simulink library "inp"  (R2021b)
settings: Solver=VariableStepAuto  StartTime=0.0  StopTime=10.0  RelTol=1e-3
undefined symbols (not defined in the file): C_TASK_5MS_S, FALSE, KINP_AcoreReadyToSlp_flg_ovrdflg, KINP_AcoreReadyToSlp_flg_ovrdval, KINP_AllowMovThd_OTA_enum_ovrdflg, KINP_AllowMovThd_OTA_enum_ovrdval, KINP_APSAngleTarget_Deg_ovrdflg, KINP_APSAngleTarget_Deg_ovrdval, KINP_APSDecReq_mps2_ovrdflg, KINP_APSDecReq_mps2_ovrdval, KINP_APSDecReqA_flg_ovrdflg, KINP_APSDecReqA_flg_ovrdval, KINP_APSDFLL_cm_ovrdflg, KINP_APSDFLL_cm_ovrdval, KINP_APSDFLR_cm_ovrdflg, KINP_APSDFLR_cm_ovrdval, KINP_APSDRLL_cm_ovrdflg, KINP_APSDRLL_cm_ovrdval, KINP_APSDRLR_cm_ovrdflg, KINP_APSDRLR_cm_ovrdval, KINP_APSExitCondition_enum_ovrdflg, KINP_APSExitCondition_enum_ovrdval, KINP_APSHWVer_enum_ovrdflg, KINP_APSHWVer_enum_ovrdval, KINP_APSProgressPCT_pct_ovrdflg, KINP_APSProgressPCT_pct_ovrdval, KINP_APSReq_enum_ovrdflg, KINP_APSReq_enum_ovrdval, KINP_APSRQDisplay_enum_ovrdflg, KINP_APSRQDisplay_enum_ovrdval, KINP_APSRqEPASCtrl_flg_ovrdflg, KINP_APSRqEPASCtrl_flg_ovrdval, KINP_APSShiftPosnReq_enum_ovrdval, KINP_APSShiftPosnReq_enum_ovrflg, KINP_APSSpeedCMD_kph_ovrdval, KINP_APSSpeedCMD_kph_ovrflg, KINP_APSStaSystem_enum_ovrdflg, KINP_APSStaSystem_enum_ovrdval, KINP_APSSWVer_enum_ovrdflg, KINP_APSSWVer_enum_ovrdval, KINP_APSVMCReqA_flg_ovrdval, KINP_APSVMCReqA_flg_ovrflg, KINP_APSVRqEPASCtrl_flg_ovrdflg, KINP_APSVRqEPASCtrl_flg_ovrdval, KINP_AuxBattVolmV_mV_ovrdflg, KINP_AuxBattVolmV_mV_ovrdval, KINP_CAASSta_enum_ovrdflg, KINP_CAASSta_enum_ovrdval, KINP_CAASVMCReqA_flg_ovrdval, KINP_CAASVMCReqA_flg_ovrflg, KINP_Chime_enum_ovrdflg, KINP_Chime_enum_ovrdval, KINP_ClearDTCcmd_flg_ovrdflg, KINP_ClearDTCcmd_flg_ovrdval, KINP_EvccAplusPwrUpReq_flg_ovrdflg, KINP_EvccAplusPwrUpReq_flg_ovrdval, KINP_LFID_raw_ovrdval, KINP_LFID_raw_ovrflg, KINP_LRID_raw_ovrdval, KINP_MemOffsetAccX_raw16_ovrdflg ... (+118)
libraries: FVT_lib x595, hcu_lib x1
(part 5 of 27)

== system inp/INP/CAN3/CommunicationCheck ==
  BHAL_outputs : Inport
  CANMsgInvalidBMS1 : FVT_lib/inp/CAN_Msg_Validity_Process_template  SystemSampleTime=-1  VariantActivationTime=update diagram  Latency=0  AutoFrameSizeCalculation=off
      link override debdec: Value=KINP_CANMsgInvalidBMS1_flg_debdec
      link override debinc: Value=KINP_CANMsgInvalidBMS1_flg_debinc
      link override deblim: Value=KINP_CANMsgInvalidBMS1_flg_deblim
      link override inverse: Value=KINP_CANMsgInvalidBMS1_flg_inverse
      link override ovrdflg: Value=KINP_CANMsgInvalidBMS1_flg_ovrdflg
      link override ovrdval: Value=KINP_CANMsgInvalidBMS1_flg_ovrdval
      link override srvcflg: Value=KINP_CANMsgInvalidBMS1_flg_srvcflg
      link override srvcval: Value=KINP_CANMsgInvalidBMS1_flg_srvcval
  CANMsgInvalidBMS2 : FVT_lib/inp/CAN_Msg_Validity_Process_template  SystemSampleTime=-1  VariantActivationTime=update diagram  Latency=0  AutoFrameSizeCalculation=off
      link override debdec: Value=KINP_CANMsgInvalidBMS2_flg_debdec
      link override debinc: Value=KINP_CANMsgInvalidBMS2_flg_debinc
      link override deblim: Value=KINP_CANMsgInvalidBMS2_flg_deblim
      link override inverse: Value=KINP_CANMsgInvalidBMS2_flg_inverse
      link override ovrdflg: Value=KINP_CANMsgInvalidBMS2_flg_ovrdflg
      link override ovrdval: Value=KINP_CANMsgInvalidBMS2_flg_ovrdval
      link override srvcflg: Value=KINP_CANMsgInvalidBMS2_flg_srvcflg
      link override srvcval: Value=KINP_CANMsgInvalidBMS2_flg_srvcval
  CANMsgInvalidBMS3 : FVT_lib/inp/CAN_Msg_Validity_Process_template  SystemSampleTime=-1  VariantActivationTime=update diagram  Latency=0  AutoFrameSizeCalculation=off
      link override debdec: Value=KINP_CANMsgInvalidBMS3_flg_debdec
      link override debinc: Value=KINP_CANMsgInvalidBMS3_flg_debinc
      link override deblim: Value=KINP_CANMsgInvalidBMS3_flg_deblim
      link override inverse: Value=KINP_CANMsgInvalidBMS3_flg_inverse
      link override ovrdflg: Value=KINP_CANMsgInvalidBMS3_flg_ovrdflg
      link override ovrdval: Value=KINP_CANMsgInvalidBMS3_flg_ovrdval
      link override srvcflg: Value=KINP_CANMsgInvalidBMS3_flg_srvcflg
      link override srvcval: Value=KINP_CANMsgInvalidBMS3_flg_srvcval
  CANMsgInvalidBMS4 : FVT_lib/inp/CAN_Msg_Validity_Process_template  SystemSampleTime=-1  VariantActivationTime=update diagram  Latency=0  AutoFrameSizeCalculation=off
      link override debdec: Value=KINP_CANMsgInvalidBMS4_flg_debdec
      link override debinc: Value=KINP_CANMsgInvalidBMS4_flg_debinc
      link override deblim: Value=KINP_CANMsgInvalidBMS4_flg_deblim
      link override inverse: Value=KINP_CANMsgInvalidBMS4_flg_inverse
      link override ovrdflg: Value=KINP_CANMsgInvalidBMS4_flg_ovrdflg
      link override ovrdval: Value=KINP_CANMsgInvalidBMS4_flg_ovrdval
      link override srvcflg: Value=KINP_CANMsgInvalidBMS4_flg_srvcflg
      link override srvcval: Value=KINP_CANMsgInvalidBMS4_flg_srvcval
  CANMsgInvalidBMS6 : FVT_lib/inp/CAN_Msg_Validity_Process_template  SystemSampleTime=-1  VariantActivationTime=update diagram  Latency=0  AutoFrameSizeCalculation=off
      link override debdec: Value=KINP_CANMsgInvalidBMS6_flg_debdec
      link override debinc: Value=KINP_CANMsgInvalidBMS6_flg_debinc
      link override deblim: Value=KINP_CANMsgInvalidBMS6_flg_deblim
      link override inverse: Value=KINP_CANMsgInvalidBMS6_flg_inverse
      link override ovrdflg: Value=KINP_CANMsgInvalidBMS6_flg_ovrdflg
      link override ovrdval: Value=KINP_CANMsgInvalidBMS6_flg_ovrdval
      link override srvcflg: Value=KINP_CANMsgInvalidBMS6_flg_srvcflg
      link override srvcval: Value=KINP_CANMsgInvalidBMS6_flg_srvcval
  CANMsgInvalidBMS7 : FVT_lib/inp/CAN_Msg_Validity_Process_template  SystemSampleTime=-1  VariantActivationTime=update diagram  Latency=0  AutoFrameSizeCalculation=off
      link override debdec: Value=KINP_CANMsgInvalidBMS7_flg_debdec
      link override debinc: Value=KINP_CANMsgInvalidBMS7_flg_debinc
      link override deblim: Value=KINP_CANMsgInvalidBMS7_flg_deblim
      link override inverse: Value=KINP_CANMsgInvalidBMS7_flg_inverse
      link override ovrdflg: Value=KINP_CANMsgInvalidBMS7_flg_ovrdflg
      link override ovrdval: Value=KINP_CANMsgInvalidBMS7_flg_ovrdval
      link override srvcflg: Value=KINP_CANMsgInvalidBMS7_flg_srvcflg
      link override srvcval: Value=KINP_CANMsgInvalidBMS7_flg_srvcval
  CANMsgInvalidCCU1 : FVT_lib/inp/CAN_Msg_Validity_Process_template  SystemSampleTime=-1  VariantActivationTime=update diagram  Latency=0  AutoFrameSizeCalculation=off
      link override debdec: Value=KINP_CANMsgInvalidCCU1_flg_debdec
      link override debinc: Value=KINP_CANMsgInvalidCCU1_flg_debinc
      link override deblim: Value=KINP_CANMsgInvalidCCU1_flg_deblim
      link override inverse: Value=KINP_CANMsgInvalidCCU1_flg_inverse
      link override ovrdflg: Value=KINP_CANMsgInvalidCCU1_flg_ovrdflg
      link override ovrdval: Value=KINP_CANMsgInvalidCCU1_flg_ovrdval
      link override srvcflg: Value=KINP_CANMsgInvalidCCU1_flg_srvcflg
      link override srvcval: Value=KINP_CANMsgInvalidCCU1_flg_srvcval
  CANMsgInvalidCCU2 : FVT_lib/inp/CAN_Msg_Validity_Process_template  SystemSampleTime=-1  VariantActivationTime=update diagram  Latency=0  AutoFrameSizeCalculation=off
      link override debdec: Value=KINP_CANMsgInvalidCCU2_flg_debdec
      link override debinc: Value=KINP_CANMsgInvalidCCU2_flg_debinc
      link override deblim: Value=KINP_CANMsgInvalidCCU2_flg_deblim
      link override inverse: Value=KINP_CANMsgInvalidCCU2_flg_inverse
      link override ovrdflg: Value=KINP_CANMsgInvalidCCU2_flg_ovrdflg
      link override ovrdval: Value=KINP_CANMsgInvalidCCU2_flg_ovrdval
      link override srvcflg: Value=KINP_CANMsgInvalidCCU2_flg_srvcflg
      link override srvcval: Value=KINP_CANMsgInvalidCCU2_flg_srvcval
  CANMsgInvalidCCU4 : FVT_lib/inp/CAN_Msg_Validity_Process_template  SystemSampleTime=-1  VariantActivationTime=update diagram  Latency=0  AutoFrameSizeCalculation=off
      link override debdec: Value=KINP_CANMsgInvalidCCU4_flg_debdec
      link override debinc: Value=KINP_CANMsgInvalidCCU4_flg_debinc
      link override deblim: Value=KINP_CANMsgInvalidCCU4_flg_deblim
      link override inverse: Value=KINP_CANMsgInvalidCCU4_flg_inverse
      link override ovrdflg: Value=KINP_CANMsgInvalidCCU4_flg_ovrdflg
      link override ovrdval: Value=KINP_CANMsgInvalidCCU4_flg_ovrdval
      link override srvcflg: Value=KINP_CANMsgInvalidCCU4_flg_srvcflg
      link override srvcval: Value=KINP_CANMsgInvalidCCU4_flg_srvcval
  CANMsgInvalidMCUF1 : FVT_lib/inp/CAN_Msg_Validity_Process_template  SystemSampleTime=-1  VariantActivationTime=update diagram  Latency=0  AutoFrameSizeCalculation=off
      link override debdec: Value=KINP_CANMsgInvalidMCUF1_flg_debdec
      link override debinc: Value=KINP_CANMsgInvalidMCUF1_flg_debinc
      link override deblim: Value=KINP_CANMsgInvalidMCUF1_flg_deblim
      link override inverse: Value=KINP_CANMsgInvalidMCUF1_flg_inverse
      link override ovrdflg: Value=KINP_CANMsgInvalidMCUF1_flg_ovrdflg
      link override ovrdval: Value=KINP_CANMsgInvalidMCUF1_flg_ovrdval
      link override srvcflg: Value=KINP_CANMsgInvalidMCUF1_flg_srvcflg
      link override srvcval: Value=KINP_CANMsgInvalidMCUF1_flg_srvcval
  CANMsgInvalidMCUF2 : FVT_lib/inp/CAN_Msg_Validity_Process_template  SystemSampleTime=-1  VariantActivationTime=update diagram  Latency=0  AutoFrameSizeCalculation=off
      link override debdec: Value=KINP_CANMsgInvalidMCUF2_flg_debdec
      link override debinc: Value=KINP_CANMsgInvalidMCUF2_flg_debinc
      link override deblim: Value=KINP_CANMsgInvalidMCUF2_flg_deblim
      link override inverse: Value=KINP_CANMsgInvalidMCUF2_flg_inverse
      link override ovrdflg: Value=KINP_CANMsgInvalidMCUF2_flg_ovrdflg
      link override ovrdval: Value=KINP_CANMsgInvalidMCUF2_flg_ovrdval
      link override srvcflg: Value=KINP_CANMsgInvalidMCUF2_flg_srvcflg
      link override srvcval: Value=KINP_CANMsgInvalidMCUF2_flg_srvcval
  CANMsgInvalidMCUR1 : FVT_lib/inp/CAN_Msg_Validity_Process_template  SystemSampleTime=-1  VariantActivationTime=update diagram  Latency=0  AutoFrameSizeCalculation=off
      link override debdec: Value=KINP_CANMsgInvalidMCUR1_flg_debdec
      link override debinc: Value=KINP_CANMsgInvalidMCUR1_flg_debinc
      link override deblim: Value=KINP_CANMsgInvalidMCUR1_flg_deblim
      link override inverse: Value=KINP_CANMsgInvalidMCUR1_flg_inverse
      link override ovrdflg: Value=KINP_CANMsgInvalidMCUR1_flg_ovrdflg
      link override ovrdval: Value=KINP_CANMsgInvalidMCUR1_flg_ovrdval
      link override srvcflg: Value=KINP_CANMsgInvalidMCUR1_flg_srvcflg
      link override srvcval: Value=KINP_CANMsgInvalidMCUR1_flg_srvcval
  CANMsgInvalidMCUR2 : FVT_lib/inp/CAN_Msg_Validity_Process_template  SystemSampleTime=-1  VariantActivationTime=update diagram  Latency=0  AutoFrameSizeCalculation=off
      link override debdec: Value=KINP_CANMsgInvalidMCUR2_flg_debdec
      link override debinc: Value=KINP_CANMsgInvalidMCUR2_flg_debinc
      link override deblim: Value=KINP_CANMsgInvalidMCUR2_flg_deblim
      link override inverse: Value=KINP_CANMsgInvalidMCUR2_flg_inverse
      link override ovrdflg: Value=KINP_CANMsgInvalidMCUR2_flg_ovrdflg
      link override ovrdval: Value=KINP_CANMsgInvalidMCUR2_flg_ovrdval
      link override srvcflg: Value=KINP_CANMsgInvalidMCUR2_flg_srvcflg
      link override srvcval: Value=KINP_CANMsgInvalidMCUR2_flg_srvcval
  CANMsgInvalidShifter1 : FVT_lib/inp/CAN_Msg_Validity_Process_template  SystemSampleTime=-1  VariantActivationTime=update diagram  Latency=0  AutoFrameSizeCalculation=off
      link override debdec: Value=KINP_CANMsgInvalidShifter1_flg_debdec
      link override debinc: Value=KINP_CANMsgInvalidShifter1_flg_debinc
      link override deblim: Value=KINP_CANMsgInvalidShifter1_flg_deblim
      link override inverse: Value=KINP_CANMsgInvalidShifter1_flg_inverse
      link override ovrdflg: Value=KINP_CANMsgInvalidShifter1_flg_ovrdflg
      link override ovrdval: Value=KINP_CANMsgInvalidShifter1_flg_ovrdval
      link override srvcflg: Value=KINP_CANMsgInvalidShifter1_flg_srvcflg
      link override srvcval: Value=KINP_CANMsgInvalidShifter1_flg_srvcval
  bus_creator : BusCreator  Inputs=14
  bus_selector : BusSelector  OutputSignals=VHAL_CANMsgInvalidBMS1_flg,VHAL_CANMsgInvalidBMS2_flg,VHAL_CANMsgInvalidBMS3_flg,VHAL_CANMsgInvalidBMS4_flg,VHAL_CANMsgInvalidBMS6_flg,VHAL_CANMsgInvalidBMS7_flg,VHAL_CANMsgInvalidCCU1_flg,VHAL_CANMsgInvalidCCU2_flg,VHAL_CANMsgInvalidCCU4_flg,VHAL_CANMsgInvalidMCUF1_flg,VHAL_CANMsgInvalidMCUF2_flg,VHAL_CANMsgInvalidMCUR1_flg,VHAL_CANMsgInvalidMCUR2_flg,VHAL_CANMsgInvalidShifter1_flg
  not{1..14} (14 alike) : Logic  Operator=NOT  AllPortsSameDT=off  OutDataTypeStr=boolean
  inp_CanValid_bus : Outport
  wires:
  BHAL_outputs/1 -> [BHAL_outputs]
  bus_selector/1 -> CANMsgInvalidBMS1/1  "<VHAL_CANMsgInvalidBMS1_flg>"
  CANMsgInvalidBMS1/1 -> not1/1
  not1/1 -> bus_creator/1  "VINP_CANMsgValidBMS1_flg"
  bus_selector/2 -> CANMsgInvalidBMS2/1  "<VHAL_CANMsgInvalidBMS2_flg>"
  CANMsgInvalidBMS2/1 -> not2/1
  not2/1 -> bus_creator/2  "VINP_CANMsgValidBMS2_flg"
  bus_selector/3 -> CANMsgInvalidBMS3/1  "<VHAL_CANMsgInvalidBMS3_flg>"
  CANMsgInvalidBMS3/1 -> not3/1
  not3/1 -> bus_creator/3  "VINP_CANMsgValidBMS3_flg"
  bus_selector/4 -> CANMsgInvalidBMS4/1  "<VHAL_CANMsgInvalidBMS4_flg>"
  CANMsgInvalidBMS4/1 -> not4/1
  not4/1 -> bus_creator/4  "VINP_CANMsgValidBMS4_flg"
  bus_selector/5 -> CANMsgInvalidBMS6/1  "<VHAL_CANMsgInvalidBMS6_flg>"
  CANMsgInvalidBMS6/1 -> not5/1
  not5/1 -> bus_creator/5  "VINP_CANMsgValidBMS6_flg"
  bus_selector/6 -> CANMsgInvalidBMS7/1  "<VHAL_CANMsgInvalidBMS7_flg>"
  CANMsgInvalidBMS7/1 -> not6/1
  not6/1 -> bus_creator/6  "VINP_CANMsgValidBMS7_flg"
  bus_selector/7 -> CANMsgInvalidCCU1/1  "<VHAL_CANMsgInvalidCCU1_flg>"
  CANMsgInvalidCCU1/1 -> not7/1
  not7/1 -> bus_creator/7  "VINP_CANMsgValidCCU1_flg"
  bus_selector/8 -> CANMsgInvalidCCU2/1  "<VHAL_CANMsgInvalidCCU2_flg>"
  CANMsgInvalidCCU2/1 -> not8/1
  not8/1 -> bus_creator/8  "VINP_CANMsgValidCCU2_flg"
  bus_selector/9 -> CANMsgInvalidCCU4/1  "<VHAL_CANMsgInvalidCCU4_flg>"
  CANMsgInvalidCCU4/1 -> not9/1
  not9/1 -> bus_creator/9  "VINP_CANMsgValidCCU4_flg"
  bus_selector/10 -> CANMsgInvalidMCUF1/1  "<VHAL_CANMsgInvalidMCUF1_flg>"
  CANMsgInvalidMCUF1/1 -> not10/1
  not10/1 -> bus_creator/10  "VINP_CANMsgValidMCUF1_flg"
  bus_selector/11 -> CANMsgInvalidMCUF2/1  "<VHAL_CANMsgInvalidMCUF2_flg>"
  CANMsgInvalidMCUF2/1 -> not11/1
  not11/1 -> bus_creator/11  "VINP_CANMsgValidMCUF2_flg"
  bus_selector/12 -> CANMsgInvalidMCUR1/1  "<VHAL_CANMsgInvalidMCUR1_flg>"
  CANMsgInvalidMCUR1/1 -> not12/1
  not12/1 -> bus_creator/12  "VINP_CANMsgValidMCUR1_flg"
  bus_selector/13 -> CANMsgInvalidMCUR2/1  "<VHAL_CANMsgInvalidMCUR2_flg>"
  CANMsgInvalidMCUR2/1 -> not13/1
  not13/1 -> bus_creator/13  "VINP_CANMsgValidMCUR2_flg"
  bus_selector/14 -> CANMsgInvalidShifter1/1  "<VHAL_CANMsgInvalidShifter1_flg>"
  CANMsgInvalidShifter1/1 -> not14/1
  not14/1 -> bus_creator/14  "VINP_CANMsgValidShifter1_flg"
  [BHAL_outputs] -> bus_selector/1
  bus_creator/1 -> inp_CanValid_bus/1

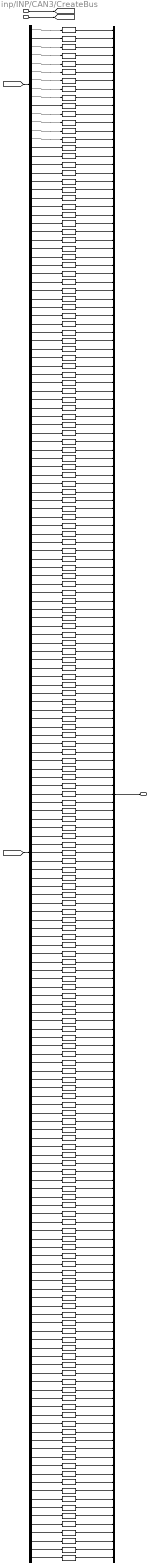
== system inp/INP/CAN3/CreateBus ==
  inp_CanValid_bus : Inport
  inp_Hal_bus : Inport  Port=2
  UnitConverter_{1..16,51..52,55..63,66..67,70,72..74,82,84..85,87,89,93,95..96,103..107,116..117,119..121,141..142,144..146,155..156,158..160,179..180} (63 alike) : DataTypeConversion  OutDataTypeStr=boolean
  UnitConverter_{17..18,47..50,53..54,64..65,68..69,71,75,78,81,83,86,88,94,98..100,109,111..112,118,122,130,133..136,139..140,143,148,150..151,157,161,171..174,177..178,181..183} (50 alike) : DataTypeConversion  OutDataTypeStr=uint8
  UnitConverter_{19..46,76..77,79..80,90..92,97,101..102,108,110,113..115,123..129,131..132,137..138,147,149,152..154,162..170,175..176} (70 alike) : DataTypeConversion  OutDataTypeStr=single
  bus_creator : BusCreator  Inputs=183
  bus_selector : BusSelector  OutputSignals=VINP_CANMsgValidBMS1_flg,VINP_CANMsgValidBMS2_flg,VINP_CANMsgValidBMS3_flg,VINP_CANMsgValidBMS4_flg,VINP_CANMsgValidBMS6_flg,VINP_CANMsgValidBMS7_flg,VINP_CANMsgValidCCU1_flg,VINP_CANMsgValidCCU2_flg,VINP_CANMsgValidCCU4_flg,VINP_CANMsgValidMCUF1_flg,VINP_CANMsgValidMCUF2_flg,VINP_CANMsgValidMCUR1_flg,VINP_CANMsgValidMCUR2_flg,VINP_CANMsgValidShifter1_flg
  bus_selector_1 : BusSelector  OutputSignals=VINP_BMS1CSErr_flg,VINP_BMS1RCErr_flg,VINP_BMSChckSum1_enum,VINP_BMSRolCnct1_enum,VINP_HVBPwrAvailChrg_kW,VINP_HVBPwrAvailChrg30_kW,VINP_HVBPwrAvailChrg60_kW,VINP_HVBPwrAvailDchrg_kW,VINP_HVBPwrAvailDchrg30_kW,VINP_HVBPwrAvailDchrg60_kW,VINP_HVInVolt_V,VINP_LVBattDet12V_V,VINP_OBCDCCurLm_A,VINP_OBCDCVoltLm_V,VINP_ACChrgCurrDis_A,VINP_HVBChrgPwr_kWh,VINP_HVBChrgPwrTotal_kWh,VINP_HVBDrvPwr_kWh,VINP_HVBDrvPwrTotal_kWh,VINP_HVBFullChrgPwr_kWh,VINP_HVBIsoImpedenceN_Megaohm,VINP_HVBIsoImpedenceP_Megaohm,VINP_HVBSOH_pct,VINP_HVBattPackVolt_V,VINP_HVBattSOC_pct,VINP_HVBattSOCDis_pct,VINP_RemainChrgTime_min,VINP_CellTempAvg_C,VINP_HVBCellVoltMax_mV,VINP_HVBCellVoltMin_mV,VINP_HVBMTempMax_C,VINP_HVBMTempMin_C,VINP_MaxCellTempNum_enum,VINP_MaxCellVoltNum_enum,VINP_MinCellTempNum_enum,VINP_MinCellVoltNum_enum,VINP_BMS6CSErr_flg,VINP_BMS6RCErr_flg,VINP_BMSChckSum_enum,VINP_BMSRolCnct_enum,VINP_BMSREADY_flg,VINP_BMSWarn1_flg,VINP_BMSWarn2_flg,VINP_BMSWarn3_flg,VINP_BMSWarn4_flg,VINP_BMSWarn5_flg,VINP_BMSWarn6_flg,VINP_BMSWarn7_flg,VINP_BMSWarn8_flg,VINP_ChrgPlugSta_enum,VINP_ExtChrgSta_enum,VINP_HVBContactorSta_flg,VINP_HVBHVILErr_flg,VINP_HVBPreheatPrecoolSta_enum,VINP_HVBattReady4Pre_enum,VINP_HVILSta_flg,VINP_V2LSta_enum,VINP_HVBattErr_flg,VINP_CCU1CSErr_flg,VINP_CCU1RCErr_flg,VINP_CSCCU1_enum,VINP_DCDCAuxVolt_V,VINP_DCDCInVoltInf_V,VINP_DCDCPreCompleted_enum,VINP_OBCDCCurrInf_A,VINP_OBCDCVoltInf_V,VINP_OBCPreCompleted_enum,VINP_OBCWakeup4Plugin_flg,VINP_RCCCU1_enum,VINP_CCU2CSErr_flg,VINP_CCU2RCErr_flg,VINP_CSCCU2_enum,VINP_DCDCEnaSta_flg,VINP_DCDCFaultSta_enum,VINP_DCDCReady4Pre_flg,VINP_DCDCTemp_C,VINP_OBCACCurrInf_A,VINP_OBCACVoltInf_V,VINP_OBCEnaSta_flg,VINP_OBCFaultSta_enum,VINP_OBCPluginSta_flg,VINP_OBCReady4Pre_flg,VINP_OBCTemp_C,VINP_OBCV2LSta_enum,VINP_OBCACCurLim_enum,VINP_RCCCU2_enum,VINP_DCDCAuxCur_A,VINP_DCDCHVCur_A,VINP_MCUF1CSErr_flg,VINP_MCUF1RCErr_flg,VINP_FrActvDmpDisabSta_flg,VINP_FrEDUDrtSta_flg,VINP_FrEDUOpratingSta_flg,VINP_FrEDURealTMTq_Nm,VINP_FrEDURotateDirction_enum,VINP_FrEDUTqReqFbk_Nm,VINP_FrMCU1Chksum_enum,VINP_FrMCU1RolCnt_enum,VINP_FrMCUBAT_V,VINP_FrMCUDCBusCurr_A,VINP_FrMCUDCBusVolt_V,VINP_FrMCUDischrgSta_flg,VINP_FrMCUEnaSta_flg,VINP_FrMCUErr_enum,VINP_FrMCUIGNsta_flg,VINP_FrMCUReady_flg,VINP_FrMCUReady4Pre_flg,VINP_FrMCUSysSta_enum,VINP_FrMCUTemp_C,VINP_FrMotorAvailTq_Nm,VINP_FrRegenAvailTq_Nm,VINP_FrTMSpd_rpm,VINP_FrTMTemp_C,VINP_FrTMid_A,VINP_FrTMiq_A,VINP_MCUWarnF_enum,VINP_FrCoolanttempReq_C,VINP_FrEOPSpdSet_rpm,VINP_FrFailcode1_enum,VINP_FrFailcode2_enum,VINP_FrFailcodehistory1_enum,VINP_FrFailcodehistory2_enum,VINP_FrLLCTemp_C,VINP_FrLLCflowReq_Lpmin,VINP_FrMCUTempWarn_enum,VINP_FrTMTempWarn_enum,VINP_MCUR1CSErr_flg,VINP_MCUR1RCErr_flg,VINP_MCUWarnR_enum,VINP_RrActvDmpDisabSta_flg,VINP_RrEDUDrtSta_flg,VINP_RrEDUOpratingSta_flg,VINP_RrEDURealTMTq_Nm,VINP_RrEDURotateDirction_enum,VINP_RrEDUTqReqFbk_Nm,VINP_RrMCU1Chksum_enum,VINP_RrMCU1RolCnt_enum,VINP_RrMCUBAT_V,VINP_RrMCUDCBusCurr_A,VINP_RrMCUDCBusVolt_V,VINP_RrMCUDischrgSta_flg,VINP_RrMCUEnaSta_flg,VINP_RrMCUErr_enum,VINP_RrMCUIGNsta_flg,VINP_RrMCUReady_flg,VINP_RrMCUReady4Pre_flg,VINP_RrMCUSysSta_enum,VINP_RrMCUTemp_C,VINP_RrMotorAvailTq_Nm,VINP_RrRegenAvailTq_Nm,VINP_RrTMSpd_rpm,VINP_RrTMTemp_C,VINP_RrTMid_A,VINP_RrTMiq_A,VINP_RrCoolanttempReq_cnt,VINP_RrEOPSpdSet_rpm,VINP_RrFailcode1_enum,VINP_RrFailcode2_enum,VINP_RrFailcodehistory1_enum,VINP_RrFailcodehistory2_enum,VINP_RrLLCTemp_C,VINP_RrLLCflowReq_Lpmin,VINP_RrMCUTempWarn_enum,VINP_RrTMTempWarn_enum,VINP_Shifter1CSErr_flg,VINP_Shifter1RCErr_flg,VINP_ShifterCRC8_enum,VINP_ShifterHandleCmd_enum,VINP_ShifterRC_enum
  BINP_outputs : Outport
  wires:
  inp_CanValid_bus/1 -> [inp_CanValid_bus]
  inp_Hal_bus/1 -> [inp_Hal_bus]
  bus_selector/1 -> UnitConverter_1/1  "<VINP_CANMsgValidBMS1_flg>"
  UnitConverter_1/1 -> bus_creator/1  "VINP_CANMsgValidBMS1_flg"
  bus_selector/2 -> UnitConverter_2/1  "<VINP_CANMsgValidBMS2_flg>"
  UnitConverter_2/1 -> bus_creator/2  "VINP_CANMsgValidBMS2_flg"
  bus_selector/3 -> UnitConverter_3/1  "<VINP_CANMsgValidBMS3_flg>"
  UnitConverter_3/1 -> bus_creator/3  "VINP_CANMsgValidBMS3_flg"
  bus_selector/4 -> UnitConverter_4/1  "<VINP_CANMsgValidBMS4_flg>"
  UnitConverter_4/1 -> bus_creator/4  "VINP_CANMsgValidBMS4_flg"
  bus_selector/5 -> UnitConverter_5/1  "<VINP_CANMsgValidBMS6_flg>"
  UnitConverter_5/1 -> bus_creator/5  "VINP_CANMsgValidBMS6_flg"
  bus_selector/6 -> UnitConverter_6/1  "<VINP_CANMsgValidBMS7_flg>"
  UnitConverter_6/1 -> bus_creator/6  "VINP_CANMsgValidBMS7_flg"
  bus_selector/7 -> UnitConverter_7/1  "<VINP_CANMsgValidCCU1_flg>"
  UnitConverter_7/1 -> bus_creator/7  "VINP_CANMsgValidCCU1_flg"
  bus_selector/8 -> UnitConverter_8/1  "<VINP_CANMsgValidCCU2_flg>"
  UnitConverter_8/1 -> bus_creator/8  "VINP_CANMsgValidCCU2_flg"
  bus_selector/9 -> UnitConverter_9/1  "<VINP_CANMsgValidCCU4_flg>"
  UnitConverter_9/1 -> bus_creator/9  "VINP_CANMsgValidCCU4_flg"
  bus_selector/10 -> UnitConverter_10/1  "<VINP_CANMsgValidMCUF1_flg>"
  UnitConverter_10/1 -> bus_creator/10  "VINP_CANMsgValidMCUF1_flg"
  bus_selector/11 -> UnitConverter_11/1  "<VINP_CANMsgValidMCUF2_flg>"
  UnitConverter_11/1 -> bus_creator/11  "VINP_CANMsgValidMCUF2_flg"
  bus_selector/12 -> UnitConverter_12/1  "<VINP_CANMsgValidMCUR1_flg>"
  UnitConverter_12/1 -> bus_creator/12  "VINP_CANMsgValidMCUR1_flg"
  bus_selector/13 -> UnitConverter_13/1  "<VINP_CANMsgValidMCUR2_flg>"
  UnitConverter_13/1 -> bus_creator/13  "VINP_CANMsgValidMCUR2_flg"
  bus_selector/14 -> UnitConverter_14/1  "<VINP_CANMsgValidShifter1_flg>"
  UnitConverter_14/1 -> bus_creator/14  "VINP_CANMsgValidShifter1_flg"
  bus_selector_1/1 -> UnitConverter_15/1  "<VINP_BMS1CSErr_flg>"
  UnitConverter_15/1 -> bus_creator/15  "VINP_BMS1CSErr_flg"
  bus_selector_1/2 -> UnitConverter_16/1  "<VINP_BMS1RCErr_flg>"
  UnitConverter_16/1 -> bus_creator/16  "VINP_BMS1RCErr_flg"
  bus_selector_1/3 -> UnitConverter_17/1  "<VINP_BMSChckSum1_enum>"
  UnitConverter_17/1 -> bus_creator/17  "VINP_BMSChckSum1_enum"
  bus_selector_1/4 -> UnitConverter_18/1  "<VINP_BMSRolCnct1_enum>"
  UnitConverter_18/1 -> bus_creator/18  "VINP_BMSRolCnct1_enum"
  bus_selector_1/5 -> UnitConverter_19/1  "<VINP_HVBPwrAvailChrg_kW>"
  UnitConverter_19/1 -> bus_creator/19  "VINP_HVBPwrAvailChrg_kW"
  bus_selector_1/6 -> UnitConverter_20/1  "<VINP_HVBPwrAvailChrg30_kW>"
  UnitConverter_20/1 -> bus_creator/20  "VINP_HVBPwrAvailChrg30_kW"
  bus_selector_1/7 -> UnitConverter_21/1  "<VINP_HVBPwrAvailChrg60_kW>"
  UnitConverter_21/1 -> bus_creator/21  "VINP_HVBPwrAvailChrg60_kW"
  bus_selector_1/8 -> UnitConverter_22/1  "<VINP_HVBPwrAvailDchrg_kW>"
  UnitConverter_22/1 -> bus_creator/22  "VINP_HVBPwrAvailDchrg_kW"
  bus_selector_1/9 -> UnitConverter_23/1  "<VINP_HVBPwrAvailDchrg30_kW>"
  UnitConverter_23/1 -> bus_creator/23  "VINP_HVBPwrAvailDchrg30_kW"
  bus_selector_1/10 -> UnitConverter_24/1  "<VINP_HVBPwrAvailDchrg60_kW>"
  UnitConverter_24/1 -> bus_creator/24  "VINP_HVBPwrAvailDchrg60_kW"
  bus_selector_1/11 -> UnitConverter_25/1  "<VINP_HVInVolt_V>"
  UnitConverter_25/1 -> bus_creator/25  "VINP_HVInVolt_V"
  bus_selector_1/12 -> UnitConverter_26/1  "<VINP_LVBattDet12V_V>"
  UnitConverter_26/1 -> bus_creator/26  "VINP_LVBattDet12V_V"
  bus_selector_1/13 -> UnitConverter_27/1  "<VINP_OBCDCCurLm_A>"
  UnitConverter_27/1 -> bus_creator/27  "VINP_OBCDCCurLm_A"
  bus_selector_1/14 -> UnitConverter_28/1  "<VINP_OBCDCVoltLm_V>"
  UnitConverter_28/1 -> bus_creator/28  "VINP_OBCDCVoltLm_V"
  bus_selector_1/15 -> UnitConverter_29/1  "<VINP_ACChrgCurrDis_A>"
  UnitConverter_29/1 -> bus_creator/29  "VINP_ACChrgCurrDis_A"
  bus_selector_1/16 -> UnitConverter_30/1  "<VINP_HVBChrgPwr_kWh>"
  UnitConverter_30/1 -> bus_creator/30  "VINP_HVBChrgPwr_kWh"
  bus_selector_1/17 -> UnitConverter_31/1  "<VINP_HVBChrgPwrTotal_kWh>"
  UnitConverter_31/1 -> bus_creator/31  "VINP_HVBChrgPwrTotal_kWh"
  bus_selector_1/18 -> UnitConverter_32/1  "<VINP_HVBDrvPwr_kWh>"
  UnitConverter_32/1 -> bus_creator/32  "VINP_HVBDrvPwr_kWh"
  bus_selector_1/19 -> UnitConverter_33/1  "<VINP_HVBDrvPwrTotal_kWh>"
  UnitConverter_33/1 -> bus_creator/33  "VINP_HVBDrvPwrTotal_kWh"
  bus_selector_1/20 -> UnitConverter_34/1  "<VINP_HVBFullChrgPwr_kWh>"
  UnitConverter_34/1 -> bus_creator/34  "VINP_HVBFullChrgPwr_kWh"
  bus_selector_1/21 -> UnitConverter_35/1  "<VINP_HVBIsoImpedenceN_Megaohm>"
  UnitConverter_35/1 -> bus_creator/35  "VINP_HVBIsoImpedenceN_Megaohm"
  bus_selector_1/22 -> UnitConverter_36/1  "<VINP_HVBIsoImpedenceP_Megaohm>"
  UnitConverter_36/1 -> bus_creator/36  "VINP_HVBIsoImpedenceP_Megaohm"
  bus_selector_1/23 -> UnitConverter_37/1  "<VINP_HVBSOH_pct>"
  UnitConverter_37/1 -> bus_creator/37  "VINP_HVBSOH_pct"
  bus_selector_1/24 -> UnitConverter_38/1  "<VINP_HVBattPackVolt_V>"
  UnitConverter_38/1 -> bus_creator/38  "VINP_HVBattPackVolt_V"
  bus_selector_1/25 -> UnitConverter_39/1  "<VINP_HVBattSOC_pct>"
  UnitConverter_39/1 -> bus_creator/39  "VINP_HVBattSOC_pct"
  bus_selector_1/26 -> UnitConverter_40/1  "<VINP_HVBattSOCDis_pct>"
  UnitConverter_40/1 -> bus_creator/40  "VINP_HVBattSOCDis_pct"
  bus_selector_1/27 -> UnitConverter_41/1  "<VINP_RemainChrgTime_min>"
  UnitConverter_41/1 -> bus_creator/41  "VINP_RemainChrgTime_min"
  bus_selector_1/28 -> UnitConverter_42/1  "<VINP_CellTempAvg_C>"
  UnitConverter_42/1 -> bus_creator/42  "VINP_CellTempAvg_C"
  bus_selector_1/29 -> UnitConverter_43/1  "<VINP_HVBCellVoltMax_mV>"
  UnitConverter_43/1 -> bus_creator/43  "VINP_HVBCellVoltMax_mV"
  bus_selector_1/30 -> UnitConverter_44/1  "<VINP_HVBCellVoltMin_mV>"
  UnitConverter_44/1 -> bus_creator/44  "VINP_HVBCellVoltMin_mV"
  bus_selector_1/31 -> UnitConverter_45/1  "<VINP_HVBMTempMax_C>"
  UnitConverter_45/1 -> bus_creator/45  "VINP_HVBMTempMax_C"
  bus_selector_1/32 -> UnitConverter_46/1  "<VINP_HVBMTempMin_C>"
  UnitConverter_46/1 -> bus_creator/46  "VINP_HVBMTempMin_C"
  bus_selector_1/33 -> UnitConverter_47/1  "<VINP_MaxCellTempNum_enum>"
  UnitConverter_47/1 -> bus_creator/47  "VINP_MaxCellTempNum_enum"
  bus_selector_1/34 -> UnitConverter_48/1  "<VINP_MaxCellVoltNum_enum>"
  UnitConverter_48/1 -> bus_creator/48  "VINP_MaxCellVoltNum_enum"
  bus_selector_1/35 -> UnitConverter_49/1  "<VINP_MinCellTempNum_enum>"
  UnitConverter_49/1 -> bus_creator/49  "VINP_MinCellTempNum_enum"
  bus_selector_1/36 -> UnitConverter_50/1  "<VINP_MinCellVoltNum_enum>"
  UnitConverter_50/1 -> bus_creator/50  "VINP_MinCellVoltNum_enum"
  bus_selector_1/37 -> UnitConverter_51/1  "<VINP_BMS6CSErr_flg>"
  UnitConverter_51/1 -> bus_creator/51  "VINP_BMS6CSErr_flg"
  bus_selector_1/38 -> UnitConverter_52/1  "<VINP_BMS6RCErr_flg>"
  UnitConverter_52/1 -> bus_creator/52  "VINP_BMS6RCErr_flg"
  bus_selector_1/39 -> UnitConverter_53/1  "<VINP_BMSChckSum_enum>"
  UnitConverter_53/1 -> bus_creator/53  "VINP_BMSChckSum_enum"
  bus_selector_1/40 -> UnitConverter_54/1  "<VINP_BMSRolCnct_enum>"
  UnitConverter_54/1 -> bus_creator/54  "VINP_BMSRolCnct_enum"
  bus_selector_1/41 -> UnitConverter_55/1  "<VINP_BMSREADY_flg>"
  UnitConverter_55/1 -> bus_creator/55  "VINP_BMSREADY_flg"
  bus_selector_1/42 -> UnitConverter_56/1  "<VINP_BMSWarn1_flg>"
  UnitConverter_56/1 -> bus_creator/56  "VINP_BMSWarn1_flg"
  bus_selector_1/43 -> UnitConverter_57/1  "<VINP_BMSWarn2_flg>"
  UnitConverter_57/1 -> bus_creator/57  "VINP_BMSWarn2_flg"
  bus_selector_1/44 -> UnitConverter_58/1  "<VINP_BMSWarn3_flg>"
  UnitConverter_58/1 -> bus_creator/58  "VINP_BMSWarn3_flg"
  bus_selector_1/45 -> UnitConverter_59/1  "<VINP_BMSWarn4_flg>"
  UnitConverter_59/1 -> bus_creator/59  "VINP_BMSWarn4_flg"
  bus_selector_1/46 -> UnitConverter_60/1  "<VINP_BMSWarn5_flg>"
  UnitConverter_60/1 -> bus_creator/60  "VINP_BMSWarn5_flg"
  bus_selector_1/47 -> UnitConverter_61/1  "<VINP_BMSWarn6_flg>"
  UnitConverter_61/1 -> bus_creator/61  "VINP_BMSWarn6_flg"
  bus_selector_1/48 -> UnitConverter_62/1  "<VINP_BMSWarn7_flg>"
  UnitConverter_62/1 -> bus_creator/62  "VINP_BMSWarn7_flg"
  bus_selector_1/49 -> UnitConverter_63/1  "<VINP_BMSWarn8_flg>"
  UnitConverter_63/1 -> bus_creator/63  "VINP_BMSWarn8_flg"
  bus_selector_1/50 -> UnitConverter_64/1  "<VINP_ChrgPlugSta_enum>"
  UnitConverter_64/1 -> bus_creator/64  "VINP_ChrgPlugSta_enum"
  bus_selector_1/51 -> UnitConverter_65/1  "<VINP_ExtChrgSta_enum>"
  UnitConverter_65/1 -> bus_creator/65  "VINP_ExtChrgSta_enum"
  bus_selector_1/52 -> UnitConverter_66/1  "<VINP_HVBContactorSta_flg>"
  UnitConverter_66/1 -> bus_creator/66  "VINP_HVBContactorSta_flg"
  bus_selector_1/53 -> UnitConverter_67/1  "<VINP_HVBHVILErr_flg>"
  UnitConverter_67/1 -> bus_creator/67  "VINP_HVBHVILErr_flg"
  bus_selector_1/54 -> UnitConverter_68/1  "<VINP_HVBPreheatPrecoolSta_enum>"
  UnitConverter_68/1 -> bus_creator/68  "VINP_HVBPreheatPrecoolSta_enum"
  bus_selector_1/55 -> UnitConverter_69/1  "<VINP_HVBattReady4Pre_enum>"
  UnitConverter_69/1 -> bus_creator/69  "VINP_HVBattReady4Pre_enum"
  bus_selector_1/56 -> UnitConverter_70/1  "<VINP_HVILSta_flg>"
  UnitConverter_70/1 -> bus_creator/70  "VINP_HVILSta_flg"
  bus_selector_1/57 -> UnitConverter_71/1  "<VINP_V2LSta_enum>"
  UnitConverter_71/1 -> bus_creator/71  "VINP_V2LSta_enum"
  bus_selector_1/58 -> UnitConverter_72/1  "<VINP_HVBattErr_flg>"
  UnitConverter_72/1 -> bus_creator/72  "VINP_HVBattErr_flg"
  bus_selector_1/59 -> UnitConverter_73/1  "<VINP_CCU1CSErr_flg>"
  UnitConverter_73/1 -> bus_creator/73  "VINP_CCU1CSErr_flg"
  bus_selector_1/60 -> UnitConverter_74/1  "<VINP_CCU1RCErr_flg>"
  UnitConverter_74/1 -> bus_creator/74  "VINP_CCU1RCErr_flg"
  bus_selector_1/61 -> UnitConverter_75/1  "<VINP_CSCCU1_enum>"
  UnitConverter_75/1 -> bus_creator/75  "VINP_CSCCU1_enum"
  bus_selector_1/62 -> UnitConverter_76/1  "<VINP_DCDCAuxVolt_V>"
  UnitConverter_76/1 -> bus_creator/76  "VINP_DCDCAuxVolt_V"
  bus_selector_1/63 -> UnitConverter_77/1  "<VINP_DCDCInVoltInf_V>"
  UnitConverter_77/1 -> bus_creator/77  "VINP_DCDCInVoltInf_V"
  bus_selector_1/64 -> UnitConverter_78/1  "<VINP_DCDCPreCompleted_enum>"
  UnitConverter_78/1 -> bus_creator/78  "VINP_DCDCPreCompleted_enum"
  bus_selector_1/65 -> UnitConverter_79/1  "<VINP_OBCDCCurrInf_A>"
  UnitConverter_79/1 -> bus_creator/79  "VINP_OBCDCCurrInf_A"
  bus_selector_1/66 -> UnitConverter_80/1  "<VINP_OBCDCVoltInf_V>"
  UnitConverter_80/1 -> bus_creator/80  "VINP_OBCDCVoltInf_V"
  bus_selector_1/67 -> UnitConverter_81/1  "<VINP_OBCPreCompleted_enum>"
  UnitConverter_81/1 -> bus_creator/81  "VINP_OBCPreCompleted_enum"
  bus_selector_1/68 -> UnitConverter_82/1  "<VINP_OBCWakeup4Plugin_flg>"
  UnitConverter_82/1 -> bus_creator/82  "VINP_OBCWakeup4Plugin_flg"
  bus_selector_1/69 -> UnitConverter_83/1  "<VINP_RCCCU1_enum>"
  UnitConverter_83/1 -> bus_creator/83  "VINP_RCCCU1_enum"
  bus_selector_1/70 -> UnitConverter_84/1  "<VINP_CCU2CSErr_flg>"
  UnitConverter_84/1 -> bus_creator/84  "VINP_CCU2CSErr_flg"
  bus_selector_1/71 -> UnitConverter_85/1  "<VINP_CCU2RCErr_flg>"
  UnitConverter_85/1 -> bus_creator/85  "VINP_CCU2RCErr_flg"
  bus_selector_1/72 -> UnitConverter_86/1  "<VINP_CSCCU2_enum>"
  UnitConverter_86/1 -> bus_creator/86  "VINP_CSCCU2_enum"
  bus_selector_1/73 -> UnitConverter_87/1  "<VINP_DCDCEnaSta_flg>"
  UnitConverter_87/1 -> bus_creator/87  "VINP_DCDCEnaSta_flg"
  bus_selector_1/74 -> UnitConverter_88/1  "<VINP_DCDCFaultSta_enum>"
  UnitConverter_88/1 -> bus_creator/88  "VINP_DCDCFaultSta_enum"
  bus_selector_1/75 -> UnitConverter_89/1  "<VINP_DCDCReady4Pre_flg>"
  UnitConverter_89/1 -> bus_creator/89  "VINP_DCDCReady4Pre_flg"
  bus_selector_1/76 -> UnitConverter_90/1  "<VINP_DCDCTemp_C>"
  UnitConverter_90/1 -> bus_creator/90  "VINP_DCDCTemp_C"
  bus_selector_1/77 -> UnitConverter_91/1  "<VINP_OBCACCurrInf_A>"
  UnitConverter_91/1 -> bus_creator/91  "VINP_OBCACCurrInf_A"
  bus_selector_1/78 -> UnitConverter_92/1  "<VINP_OBCACVoltInf_V>"
  UnitConverter_92/1 -> bus_creator/92  "VINP_OBCACVoltInf_V"
  bus_selector_1/79 -> UnitConverter_93/1  "<VINP_OBCEnaSta_flg>"
  UnitConverter_93/1 -> bus_creator/93  "VINP_OBCEnaSta_flg"
  bus_selector_1/80 -> UnitConverter_94/1  "<VINP_OBCFaultSta_enum>"
  UnitConverter_94/1 -> bus_creator/94  "VINP_OBCFaultSta_enum"
  bus_selector_1/81 -> UnitConverter_95/1  "<VINP_OBCPluginSta_flg>"
  UnitConverter_95/1 -> bus_creator/95  "VINP_OBCPluginSta_flg"
  bus_selector_1/82 -> UnitConverter_96/1  "<VINP_OBCReady4Pre_flg>"
  UnitConverter_96/1 -> bus_creator/96  "VINP_OBCReady4Pre_flg"
  bus_selector_1/83 -> UnitConverter_97/1  "<VINP_OBCTemp_C>"
  UnitConverter_97/1 -> bus_creator/97  "VINP_OBCTemp_C"
  bus_selector_1/84 -> UnitConverter_98/1  "<VINP_OBCV2LSta_enum>"
  UnitConverter_98/1 -> bus_creator/98  "VINP_OBCV2LSta_enum"
  bus_selector_1/85 -> UnitConverter_99/1  "<VINP_OBCACCurLim_enum>"
  UnitConverter_99/1 -> bus_creator/99  "VINP_OBCACCurLim_enum"
  bus_selector_1/86 -> UnitConverter_100/1  "<VINP_RCCCU2_enum>"
  UnitConverter_100/1 -> bus_creator/100  "VINP_RCCCU2_enum"
  bus_selector_1/87 -> UnitConverter_101/1  "<VINP_DCDCAuxCur_A>"
  UnitConverter_101/1 -> bus_creator/101  "VINP_DCDCAuxCur_A"
  bus_selector_1/88 -> UnitConverter_102/1  "<VINP_DCDCHVCur_A>"
  UnitConverter_102/1 -> bus_creator/102  "VINP_DCDCHVCur_A"
  bus_selector_1/89 -> UnitConverter_103/1  "<VINP_MCUF1CSErr_flg>"
  UnitConverter_103/1 -> bus_creator/103  "VINP_MCUF1CSErr_flg"
  bus_selector_1/90 -> UnitConverter_104/1  "<VINP_MCUF1RCErr_flg>"
  UnitConverter_104/1 -> bus_creator/104  "VINP_MCUF1RCErr_flg"
  bus_selector_1/91 -> UnitConverter_105/1  "<VINP_FrActvDmpDisabSta_flg>"
  UnitConverter_105/1 -> bus_creator/105  "VINP_FrActvDmpDisabSta_flg"
  bus_selector_1/92 -> UnitConverter_106/1  "<VINP_FrEDUDrtSta_flg>"
  UnitConverter_106/1 -> bus_creator/106  "VINP_FrEDUDrtSta_flg"
  bus_selector_1/93 -> UnitConverter_107/1  "<VINP_FrEDUOpratingSta_flg>"
  UnitConverter_107/1 -> bus_creator/107  "VINP_FrEDUOpratingSta_flg"
  bus_selector_1/94 -> UnitConverter_108/1  "<VINP_FrEDURealTMTq_Nm>"
  UnitConverter_108/1 -> bus_creator/108  "VINP_FrEDURealTMTq_Nm"
  bus_selector_1/95 -> UnitConverter_109/1  "<VINP_FrEDURotateDirction_enum>"
  UnitConverter_109/1 -> bus_creator/109  "VINP_FrEDURotateDirction_enum"
  bus_selector_1/96 -> UnitConverter_110/1  "<VINP_FrEDUTqReqFbk_Nm>"
  UnitConverter_110/1 -> bus_creator/110  "VINP_FrEDUTqReqFbk_Nm"
  bus_selector_1/97 -> UnitConverter_111/1  "<VINP_FrMCU1Chksum_enum>"
  UnitConverter_111/1 -> bus_creator/111  "VINP_FrMCU1Chksum_enum"
  bus_selector_1/98 -> UnitConverter_112/1  "<VINP_FrMCU1RolCnt_enum>"
  UnitConverter_112/1 -> bus_creator/112  "VINP_FrMCU1RolCnt_enum"
  bus_selector_1/99 -> UnitConverter_113/1  "<VINP_FrMCUBAT_V>"
  UnitConverter_113/1 -> bus_creator/113  "VINP_FrMCUBAT_V"
  bus_selector_1/100 -> UnitConverter_114/1  "<VINP_FrMCUDCBusCurr_A>"
  UnitConverter_114/1 -> bus_creator/114  "VINP_FrMCUDCBusCurr_A"
  bus_selector_1/101 -> UnitConverter_115/1  "<VINP_FrMCUDCBusVolt_V>"
  UnitConverter_115/1 -> bus_creator/115  "VINP_FrMCUDCBusVolt_V"
  bus_selector_1/102 -> UnitConverter_116/1  "<VINP_FrMCUDischrgSta_flg>"
  UnitConverter_116/1 -> bus_creator/116  "VINP_FrMCUDischrgSta_flg"
  bus_selector_1/103 -> UnitConverter_117/1  "<VINP_FrMCUEnaSta_flg>"
  UnitConverter_117/1 -> bus_creator/117  "VINP_FrMCUEnaSta_flg"
  bus_selector_1/104 -> UnitConverter_118/1  "<VINP_FrMCUErr_enum>"
  UnitConverter_118/1 -> bus_creator/118  "VINP_FrMCUErr_enum"
  bus_selector_1/105 -> UnitConverter_119/1  "<VINP_FrMCUIGNsta_flg>"
  UnitConverter_119/1 -> bus_creator/119  "VINP_FrMCUIGNsta_flg"
  bus_selector_1/106 -> UnitConverter_120/1  "<VINP_FrMCUReady_flg>"
  UnitConverter_120/1 -> bus_creator/120  "VINP_FrMCUReady_flg"
  bus_selector_1/107 -> UnitConverter_121/1  "<VINP_FrMCUReady4Pre_flg>"
  UnitConverter_121/1 -> bus_creator/121  "VINP_FrMCUReady4Pre_flg"
  bus_selector_1/108 -> UnitConverter_122/1  "<VINP_FrMCUSysSta_enum>"
  UnitConverter_122/1 -> bus_creator/122  "VINP_FrMCUSysSta_enum"
  bus_selector_1/109 -> UnitConverter_123/1  "<VINP_FrMCUTemp_C>"
  UnitConverter_123/1 -> bus_creator/123  "VINP_FrMCUTemp_C"
  bus_selector_1/110 -> UnitConverter_124/1  "<VINP_FrMotorAvailTq_Nm>"
  UnitConverter_124/1 -> bus_creator/124  "VINP_FrMotorAvailTq_Nm"
  bus_selector_1/111 -> UnitConverter_125/1  "<VINP_FrRegenAvailTq_Nm>"
  UnitConverter_125/1 -> bus_creator/125  "VINP_FrRegenAvailTq_Nm"
  bus_selector_1/112 -> UnitConverter_126/1  "<VINP_FrTMSpd_rpm>"
  UnitConverter_126/1 -> bus_creator/126  "VINP_FrTMSpd_rpm"
  bus_selector_1/113 -> UnitConverter_127/1  "<VINP_FrTMTemp_C>"
  UnitConverter_127/1 -> bus_creator/127  "VINP_FrTMTemp_C"
  bus_selector_1/114 -> UnitConverter_128/1  "<VINP_FrTMid_A>"
  UnitConverter_128/1 -> bus_creator/128  "VINP_FrTMid_A"
  bus_selector_1/115 -> UnitConverter_129/1  "<VINP_FrTMiq_A>"
  UnitConverter_129/1 -> bus_creator/129  "VINP_FrTMiq_A"
  bus_selector_1/116 -> UnitConverter_130/1  "<VINP_MCUWarnF_enum>"
  UnitConverter_130/1 -> bus_creator/130  "VINP_MCUWarnF_enum"
  bus_selector_1/117 -> UnitConverter_131/1  "<VINP_FrCoolanttempReq_C>"
  UnitConverter_131/1 -> bus_creator/131  "VINP_FrCoolanttempReq_C"
  bus_selector_1/118 -> UnitConverter_132/1  "<VINP_FrEOPSpdSet_rpm>"
  UnitConverter_132/1 -> bus_creator/132  "VINP_FrEOPSpdSet_rpm"
  bus_selector_1/119 -> UnitConverter_133/1  "<VINP_FrFailcode1_enum>"
  UnitConverter_133/1 -> bus_creator/133  "VINP_FrFailcode1_enum"
  bus_selector_1/120 -> UnitConverter_134/1  "<VINP_FrFailcode2_enum>"
  UnitConverter_134/1 -> bus_creator/134  "VINP_FrFailcode2_enum"
  bus_selector_1/121 -> UnitConverter_135/1  "<VINP_FrFailcodehistory1_enum>"
  UnitConverter_135/1 -> bus_creator/135  "VINP_FrFailcodehistory1_enum"
  bus_selector_1/122 -> UnitConverter_136/1  "<VINP_FrFailcodehistory2_enum>"
  UnitConverter_136/1 -> bus_creator/136  "VINP_FrFailcodehistory2_enum"
  bus_selector_1/123 -> UnitConverter_137/1  "<VINP_FrLLCTemp_C>"
  UnitConverter_137/1 -> bus_creator/137  "VINP_FrLLCTemp_C"
  bus_selector_1/124 -> UnitConverter_138/1  "<VINP_FrLLCflowReq_Lpmin>"
  UnitConverter_138/1 -> bus_creator/138  "VINP_FrLLCflowReq_Lpmin"
  bus_selector_1/125 -> UnitConverter_139/1  "<VINP_FrMCUTempWarn_enum>"
  UnitConverter_139/1 -> bus_creator/139  "VINP_FrMCUTempWarn_enum"
  bus_selector_1/126 -> UnitConverter_140/1  "<VINP_FrTMTempWarn_enum>"
  UnitConverter_140/1 -> bus_creator/140  "VINP_FrTMTempWarn_enum"
  bus_selector_1/127 -> UnitConverter_141/1  "<VINP_MCUR1CSErr_flg>"
  UnitConverter_141/1 -> bus_creator/141  "VINP_MCUR1CSErr_flg"
  bus_selector_1/128 -> UnitConverter_142/1  "<VINP_MCUR1RCErr_flg>"
  UnitConverter_142/1 -> bus_creator/142  "VINP_MCUR1RCErr_flg"
  bus_selector_1/129 -> UnitConverter_143/1  "<VINP_MCUWarnR_enum>"
  UnitConverter_143/1 -> bus_creator/143  "VINP_MCUWarnR_enum"
  bus_selector_1/130 -> UnitConverter_144/1  "<VINP_RrActvDmpDisabSta_flg>"
  UnitConverter_144/1 -> bus_creator/144  "VINP_RrActvDmpDisabSta_flg"
  bus_selector_1/131 -> UnitConverter_145/1  "<VINP_RrEDUDrtSta_flg>"
  UnitConverter_145/1 -> bus_creator/145  "VINP_RrEDUDrtSta_flg"
  bus_selector_1/132 -> UnitConverter_146/1  "<VINP_RrEDUOpratingSta_flg>"
  UnitConverter_146/1 -> bus_creator/146  "VINP_RrEDUOpratingSta_flg"
  bus_selector_1/133 -> UnitConverter_147/1  "<VINP_RrEDURealTMTq_Nm>"
  UnitConverter_147/1 -> bus_creator/147  "VINP_RrEDURealTMTq_Nm"
  bus_selector_1/134 -> UnitConverter_148/1  "<VINP_RrEDURotateDirction_enum>"
  UnitConverter_148/1 -> bus_creator/148  "VINP_RrEDURotateDirction_enum"
  bus_selector_1/135 -> UnitConverter_149/1  "<VINP_RrEDUTqReqFbk_Nm>"
  UnitConverter_149/1 -> bus_creator/149  "VINP_RrEDUTqReqFbk_Nm"
  bus_selector_1/136 -> UnitConverter_150/1  "<VINP_RrMCU1Chksum_enum>"
  UnitConverter_150/1 -> bus_creator/150  "VINP_RrMCU1Chksum_enum"
  bus_selector_1/137 -> UnitConverter_151/1  "<VINP_RrMCU1RolCnt_enum>"
  UnitConverter_151/1 -> bus_creator/151  "VINP_RrMCU1RolCnt_enum"
  bus_selector_1/138 -> UnitConverter_152/1  "<VINP_RrMCUBAT_V>"
  UnitConverter_152/1 -> bus_creator/152  "VINP_RrMCUBAT_V"
  bus_selector_1/139 -> UnitConverter_153/1  "<VINP_RrMCUDCBusCurr_A>"
  UnitConverter_153/1 -> bus_creator/153  "VINP_RrMCUDCBusCurr_A"
  bus_selector_1/140 -> UnitConverter_154/1  "<VINP_RrMCUDCBusVolt_V>"
  UnitConverter_154/1 -> bus_creator/154  "VINP_RrMCUDCBusVolt_V"
  bus_selector_1/141 -> UnitConverter_155/1  "<VINP_RrMCUDischrgSta_flg>"
  UnitConverter_155/1 -> bus_creator/155  "VINP_RrMCUDischrgSta_flg"
  bus_selector_1/142 -> UnitConverter_156/1  "<VINP_RrMCUEnaSta_flg>"
  UnitConverter_156/1 -> bus_creator/156  "VINP_RrMCUEnaSta_flg"
  bus_selector_1/143 -> UnitConverter_157/1  "<VINP_RrMCUErr_enum>"
  UnitConverter_157/1 -> bus_creator/157  "VINP_RrMCUErr_enum"
  bus_selector_1/144 -> UnitConverter_158/1  "<VINP_RrMCUIGNsta_flg>"
  UnitConverter_158/1 -> bus_creator/158  "VINP_RrMCUIGNsta_flg"
  bus_selector_1/145 -> UnitConverter_159/1  "<VINP_RrMCUReady_flg>"
  UnitConverter_159/1 -> bus_creator/159  "VINP_RrMCUReady_flg"
  bus_selector_1/146 -> UnitConverter_160/1  "<VINP_RrMCUReady4Pre_flg>"
  UnitConverter_160/1 -> bus_creator/160  "VINP_RrMCUReady4Pre_flg"
  bus_selector_1/147 -> UnitConverter_161/1  "<VINP_RrMCUSysSta_enum>"
  UnitConverter_161/1 -> bus_creator/161  "VINP_RrMCUSysSta_enum"
  bus_selector_1/148 -> UnitConverter_162/1  "<VINP_RrMCUTemp_C>"
  UnitConverter_162/1 -> bus_creator/162  "VINP_RrMCUTemp_C"
  bus_selector_1/149 -> UnitConverter_163/1  "<VINP_RrMotorAvailTq_Nm>"
  UnitConverter_163/1 -> bus_creator/163  "VINP_RrMotorAvailTq_Nm"
  bus_selector_1/150 -> UnitConverter_164/1  "<VINP_RrRegenAvailTq_Nm>"
  UnitConverter_164/1 -> bus_creator/164  "VINP_RrRegenAvailTq_Nm"
  bus_selector_1/151 -> UnitConverter_165/1  "<VINP_RrTMSpd_rpm>"
  UnitConverter_165/1 -> bus_creator/165  "VINP_RrTMSpd_rpm"
  bus_selector_1/152 -> UnitConverter_166/1  "<VINP_RrTMTemp_C>"
  UnitConverter_166/1 -> bus_creator/166  "VINP_RrTMTemp_C"
  bus_selector_1/153 -> UnitConverter_167/1  "<VINP_RrTMid_A>"
  UnitConverter_167/1 -> bus_creator/167  "VINP_RrTMid_A"
  bus_selector_1/154 -> UnitConverter_168/1  "<VINP_RrTMiq_A>"
  UnitConverter_168/1 -> bus_creator/168  "VINP_RrTMiq_A"
  bus_selector_1/155 -> UnitConverter_169/1  "<VINP_RrCoolanttempReq_cnt>"
  UnitConverter_169/1 -> bus_creator/169  "VINP_RrCoolanttempReq_cnt"
  bus_selector_1/156 -> UnitConverter_170/1  "<VINP_RrEOPSpdSet_rpm>"
  UnitConverter_170/1 -> bus_creator/170  "VINP_RrEOPSpdSet_rpm"
  bus_selector_1/157 -> UnitConverter_171/1  "<VINP_RrFailcode1_enum>"
  UnitConverter_171/1 -> bus_creator/171  "VINP_RrFailcode1_enum"
  bus_selector_1/158 -> UnitConverter_172/1  "<VINP_RrFailcode2_enum>"
  UnitConverter_172/1 -> bus_creator/172  "VINP_RrFailcode2_enum"
  bus_selector_1/159 -> UnitConverter_173/1  "<VINP_RrFailcodehistory1_enum>"
  UnitConverter_173/1 -> bus_creator/173  "VINP_RrFailcodehistory1_enum"
  bus_selector_1/160 -> UnitConverter_174/1  "<VINP_RrFailcodehistory2_enum>"
  UnitConverter_174/1 -> bus_creator/174  "VINP_RrFailcodehistory2_enum"
  bus_selector_1/161 -> UnitConverter_175/1  "<VINP_RrLLCTemp_C>"
  UnitConverter_175/1 -> bus_creator/175  "VINP_RrLLCTemp_C"
  bus_selector_1/162 -> UnitConverter_176/1  "<VINP_RrLLCflowReq_Lpmin>"
  UnitConverter_176/1 -> bus_creator/176  "VINP_RrLLCflowReq_Lpmin"
  bus_selector_1/163 -> UnitConverter_177/1  "<VINP_RrMCUTempWarn_enum>"
  UnitConverter_177/1 -> bus_creator/177  "VINP_RrMCUTempWarn_enum"
  bus_selector_1/164 -> UnitConverter_178/1  "<VINP_RrTMTempWarn_enum>"
  UnitConverter_178/1 -> bus_creator/178  "VINP_RrTMTempWarn_enum"
  bus_selector_1/165 -> UnitConverter_179/1  "<VINP_Shifter1CSErr_flg>"
  UnitConverter_179/1 -> bus_creator/179  "VINP_Shifter1CSErr_flg"
  bus_selector_1/166 -> UnitConverter_180/1  "<VINP_Shifter1RCErr_flg>"
  UnitConverter_180/1 -> bus_creator/180  "VINP_Shifter1RCErr_flg"
  bus_selector_1/167 -> UnitConverter_181/1  "<VINP_ShifterCRC8_enum>"
  UnitConverter_181/1 -> bus_creator/181  "VINP_ShifterCRC8_enum"
  bus_selector_1/168 -> UnitConverter_182/1  "<VINP_ShifterHandleCmd_enum>"
  UnitConverter_182/1 -> bus_creator/182  "VINP_ShifterHandleCmd_enum"
  bus_selector_1/169 -> UnitConverter_183/1  "<VINP_ShifterRC_enum>"
  UnitConverter_183/1 -> bus_creator/183  "VINP_ShifterRC_enum"
  [inp_CanValid_bus] -> bus_selector/1
  [inp_Hal_bus] -> bus_selector_1/1
  bus_creator/1 -> BINP_outputs/1
